simulink library "input_system"  (R2023b)
settings: Solver=VariableStepAuto  StartTime=0.0  StopTime=10.0  RelTol=1e-3
libraries: adc_converter x1, two_state_button x1
settings Model: Creator=mueller.chris-it22  LastModifiedBy=kilia

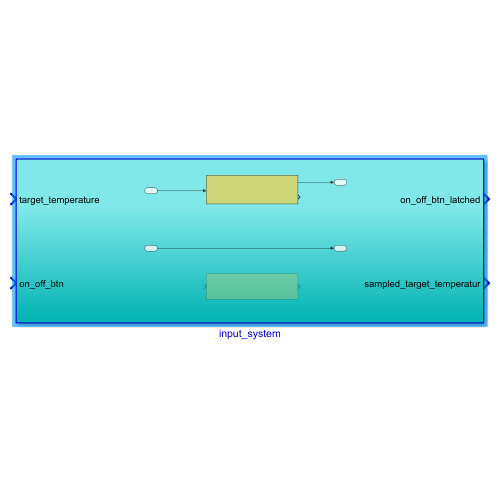
[thumbnail: Simulink's stored preview of the top-level diagram]
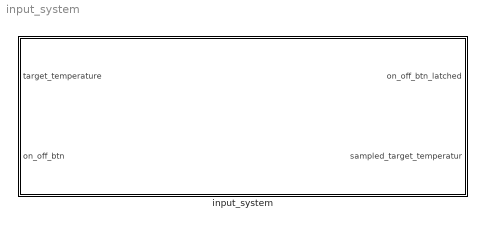
== system input_system ==
  input_system : Subsystem

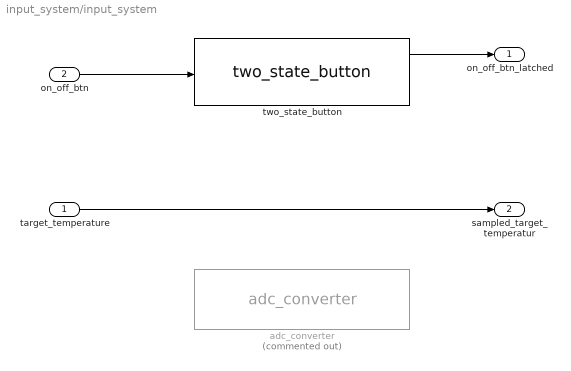
== system input_system/input_system ==
  target_temperature : Inport  OutDataTypeStr=uint16
  on_off_btn : Inport  Port=2
  adc_converter : adc_converter/adc_converter  Commented=on  SystemSampleTime=-1  VariantActivationTime=update diagram  AllowFlexibleInterface=on  Latency=0  AutoFrameSizeCalculation=off
  two_state_button : two_state_button/two_state_button  SystemSampleTime=-1  VariantActivationTime=update diagram  AllowFlexibleInterface=on  Latency=0  AutoFrameSizeCalculation=off
  on_off_btn_latched : Outport
  sampled_target_temperatur : Outport  Port=2  OutDataTypeStr=uint16
  wires:
  on_off_btn/1 -> two_state_button/1
  two_state_button/1 -> on_off_btn_latched/1
  target_temperature/1 -> sampled_target_temperatur/1
